simulink model "GolfSwing - Copy"  (R2024b)
settings: Solver=VariableStepAuto  StartTime=0.0  StopTime=StopTime  MaxStep=0.001  RelTol=1e-3
PreLoadFcn:
  | cd(matlabdrive);
  | cd '2DModel';
PostLoadFcn:
  | %run SCRIPT_mdlWksGenerate.m;
  | mdlWks=get_param('GolfSwing','ModelWorkspace');
  | mdlWks.DataSource = 'MAT-File';
  | mdlWks.FileName = 'ModelInputs.mat';
  | mdlWks.reload;
model workspace: external: MAT-File ModelInputs.mat (data not in the file)
undefined symbols (not defined in the file or in its folder): GlobalGain, HipConstant, HipDampening, HipTimeGain, KillDampFinalValue, KillDampInitialValue, KillswitchFinalValue, KillswitchInitialValue, KillswitchStepTime, LElbowConstant, LElbowDampening, LElbowTimeGain, LScapConstant, LScapDampening, LScapPositionGain, LScapTimeGain, LShoulderConstant, LShoulderDampening, LShoulderTimeGain, LWristConstant, LWristDampening, LWristTimeGain, RElbowConstant, RElbowDampening, RElbowTimeGain, RScapConstant, RScapDampening, RScapPositionGain, RScapTimeGain, RShoulderConstant, RShoulderDampening, RShoulderTimeGain, RWristConstant, RWristDampening, RWristTimeGain, TorsoConstant, TorsoDampening, TorsoPositionGain, TorsoTimeGain, WristGain, X, Y, Z
libraries: nesl_utility x204, sm_lib x102, matrix_library x11, simulink_extras x2, simulink x1
(part 6 of 6)

== matlab function GolfSwing - Copy/Club/Impact Model/Golf Ball Reaction Force ==
  data: u input; FImpact output
function FImpact = fcn(u)

FImpact=-u*1.5*.44704*.0459/.0005;
%Impact Time = 0.0005 s
%Golf Ball Mass = 0.0459 g
%MPH to m/s conversion = 0.44704 m/s / MPH
%Smash Factor = 1.5

== matlab function GolfSwing - Copy/Club/Clubhead Air Resistance Calculator/Drag Function ==
  data: u input; FDrag output
function FDrag = fcn(u)

FDrag = -1/2*1.225*3.1415927*(2.5/39)^2*0.47*u^2;
%Shape Factor = 0.47
%Air Density = 1.225 kg/m3
%CH Radius = 2.5"
%Fd=-1/2*Density*ShapeFactor*CSA*v^2

== matlab function GolfSwing - Copy/RJM Inputs/Hip Input Torque ==
  data: Time input; HipTimeGain input; JointTorqueHips output; HipConstant input; HipVelocity input; HipDamper input; Killswitch input; GlobalGain input; KillDamp input
% Time factor has been changed to depend on t^2 rather than t to get more
% drop off with time.

function JointTorqueHips = fcn(Time,HipTimeGain,HipConstant,HipVelocity,HipDamper,Killswitch,GlobalGain,KillDamp)
JointTorqueHips=Killswitch*GlobalGain*(HipTimeGain*Time+HipConstant)-GlobalGain*KillDamp*HipVelocity*HipDamper;

== matlab function GolfSwing - Copy/RJM Inputs/Torso Input Torque ==
  data: Time input; TorsoTimeGain input; JointTorqueTorso output; TorsoConstant input; TorsoVelocity input; TorsoDamper input; TorsoPosition input; TorsoPositionGain input; Killswitch input; GlobalGain input; KillDamp input
function JointTorqueTorso = fcn(Time,TorsoTimeGain,TorsoConstant,TorsoVelocity,TorsoDamper,TorsoPosition,TorsoPositionGain,Killswitch,GlobalGain,KillDamp)
JointTorqueTorso = Killswitch*GlobalGain*(TorsoTimeGain*Time+TorsoConstant-TorsoPositionGain*TorsoPosition)-GlobalGain*KillDamp*TorsoVelocity*TorsoDamper;

== matlab function GolfSwing - Copy/RJM Inputs/LScap Input Torque ==
  data: Time input; LScapTimeGain input; JointTorqueLScap output; LScapConstant input; LScapVelocity input; LScapDamper input; LScapPosition input; LScapPositionGain input; Killswitch input; GlobalGain input; KillDamp input
function JointTorqueLScap = fcn(Time,LScapTimeGain,LScapConstant,LScapVelocity,LScapDamper,LScapPosition,LScapPositionGain,Killswitch,GlobalGain,KillDamp)

% Scapula Excluded Scapula Damper Excluded in Killswitch:
JointTorqueLScap=GlobalGain*(LScapTimeGain*Time+LScapConstant-LScapPositionGain*LScapPosition)-GlobalGain*LScapVelocity*LScapDamper;

% Scapula Included Damper Included in Killswitch
%JointTorqueLScap=GlobalGain*Killswitch*(LScapTimeGain*Time+LScapConstant-LScapPositionGain*LScapPosition)-GlobalGain*KillDamp*LScapVelocity*LScapDamper;

% Scapula Excluded Damper Included in Killswitch
% JointTorqueRScap=GlobalGain*(LScapTimeGain*Time+LScapConstant-LScapPositionGain*LScapPosition)-GlobalGain*KillDamp*LScapVelocity*LScapDamper;

== matlab function GolfSwing - Copy/RJM Inputs/RScap Input Torque ==
  data: Time input; RScapTimeGain input; JointTorqueRScap output; RScapConstant input; RScapVelocity input; RScapDamper input; RScapPosition input; RScapPositionGain input; Killswitch input; GlobalGain input; KillDamp input
function JointTorqueRScap = fcn(Time,RScapTimeGain,RScapConstant,RScapVelocity,RScapDamper,RScapPosition,RScapPositionGain,Killswitch,GlobalGain,KillDamp)

% Scapula Excluded in Killswitch Scapula Damper Excluded in Killswitch
JointTorqueRScap = GlobalGain*(RScapTimeGain*Time+RScapConstant-RScapPositionGain*RScapPosition)-GlobalGain*RScapVelocity*RScapDamper;

% Scapula Included in Killswitch, Damper Included in Killswitch
%JointTorqueRScap = GlobalGain*Killswitch*(RScapTimeGain*Time+RScapConstant-RScapPositionGain*RScapPosition)-GlobalGain*KillDamp*RScapVelocity*RScapDamper;

% Scapula Excluded in Killswitch, Damper Included in Killswitch
% JointTorqueRScap = GlobalGain*(RScapTimeGain*Time+RScapConstant-RScapPositionGain*RScapPosition)-GlobalGain*KillDamp*RScapVelocity*RScapDamper;
